simulink model "stepResponseDDR"  (R2021a)
settings: Solver=VariableStepAuto  StartTime=0.0  StopTime=20  RelTol=1e-3
model workspace (MAT data in the model file):
  Velocity = 2
  axleLength = 0.1
  radius = 0.02
libraries: simulink x2, robotmobilelib x1, pid_lib x1
settings Model: NumberOfSteps=10  EnablePacing=on  PacingRate=6  Creator=yellu  LastModifiedBy=yellu

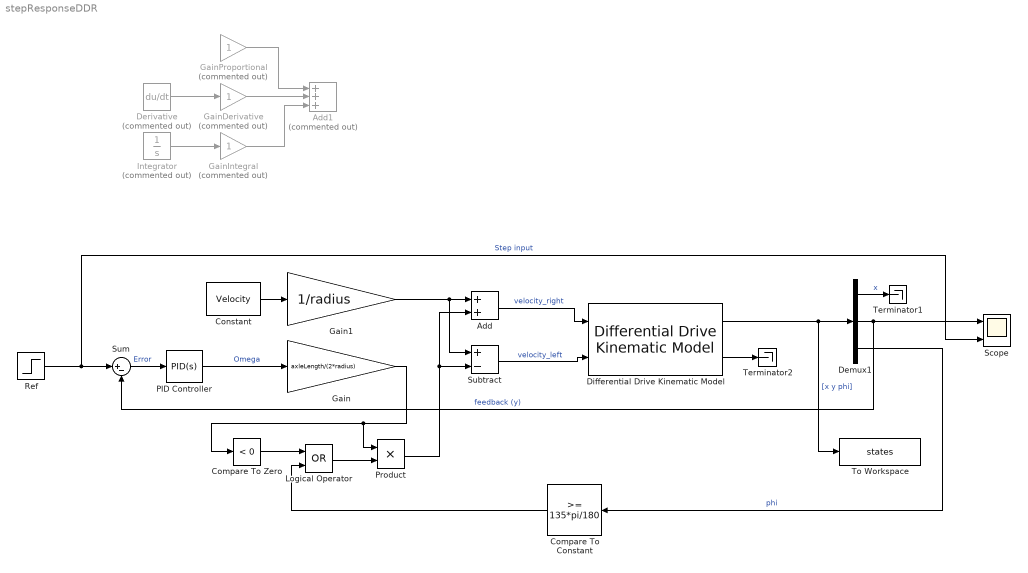
== system stepResponseDDR ==
  Add : Sum
  Add1 : Sum  Commented=on  Inputs=+++
  Compare To Constant : simulink/Logic and Bit Operations/Compare To Constant  relop=>=  const=135*pi/180  OutDataTypeStr=boolean
  Compare To Zero : simulink/Logic and Bit Operations/Compare To Zero  relop=<  OutDataTypeStr=boolean
  Constant : Constant  Value=Velocity
  Demux1 : Demux  Outputs=3
  Derivative : Derivative  Commented=on
  Differential Drive Kinematic Model : robotmobilelib/Differential Drive Kinematic Model  VehicleInputs=Wheel Speeds  WheelRadius=radius  WheelSpeedRange=[-inf inf]  TrackWidth=axleLength  InitialState=[0 0 180*pi/180]  SimulateUsing=Interpreted execution
      settings: SourceProductBaseCode=RO
  Gain : Gain  Gain=axleLength/(2*radius)
  Gain1 : Gain  Gain=1/radius
  GainDerivative : Gain  Commented=on
  GainIntegral : Gain  Commented=on
  GainProportional : Gain  Commented=on
  Integrator : Integrator  Commented=on
  Logical Operator : Logic  Operator=OR  AllPortsSameDT=off  OutDataTypeStr=boolean
  PID Controller : pid_lib/PID Controller  Controller=PID  Form=Parallel  TimeDomain=Continuous-time  UseExternalTs=off  SampleTime=-1  IntegratorMethod=Forward Euler  FilterMethod=Forward Euler  ControllerParametersSource=internal  P=0.5  I=0  D=0.8  UseFilter=on  N=100  TunerSelectOption=Transfer Function Based (PID Tuner App)  InitialConditionSource=internal  InitialConditionForIntegrator=0  InitialConditionForFilter=0  DifferentiatorICPrevScaledInput=0  ExternalReset=none  TrackingMode=off  Kt=1  LimitOutput=on  SatLimitsSource=internal  UpperSaturationLimit=4.48  LowerSaturationLimit=-4.48  LinearizeAsGain=on  AntiWindupMode=clamping  Kb=1  POutMin=[]  POutMax=[]  IOutMin=[]  IOutMax=[]  DOutMin=[]  DOutMax=[]  NOutMin=[]  NOutMax=[]  SumOutMin=[]  SumOutMax=[]  SaturationOutMin=[]  SaturationOutMax=[]  PParamMin=[]  PParamMax=[]  IParamMin=[]  IParamMax=[]  DParamMin=[]  DParamMax=[]  NParamMin=[]  NParamMax=[]  KbParamMin=[]  KbParamMax=[]  KtParamMin=[]  KtParamMax=[]  KbOutMin=[]  KbOutMax=[]  KtOutMin=[]  KtOutMax=[]  IntegratorOutMin=[]  IntegratorOutMax=[]  FilterOutMin=[]  FilterOutMax=[]  SumI1OutMin=[]  SumI1OutMax=[]  SumI2OutMin=[]  SumI2OutMax=[]  SumI3OutMin=[]  SumI3OutMax=[]  SumI4OutMin=[]  SumI4OutMax=[]  SumDOutMin=[]  SumDOutMax=[]  DifferentiatorOutMin=[]  DifferentiatorOutMax=[]  FilterDiffOutCoefMin=[]  FilterDiffOutCoefMax=[]  ReciprocalOutMin=[]  ReciprocalOutMax=[]  SumDenOutMin=[]  SumDenOutMax=[]  SumNumOutMin=[]  SumNumOutMax=[]  DivideOutMin=[]  DivideOutMax=[]  UdiffTsProdOutMin=[]  UdiffTsProdOutMax=[]  NTsProdOutMin=[]  NTsProdOutMax=[]  UintegralTsProdOutMin=[]  UintegralTsProdOutMax=[]  UngainTsProdOutMin=[]  UngainTsProdOutMax=[]  IntegratorContinuousStateAttributes=''  IntegratorStateMustResolveToSignalObject=off  IntegratorRTWStateStorageClass=Auto  FilterContinuousStateAttributes=''  FilterStateMustResolveToSignalObject=off  FilterRTWStateStorageClass=Auto  ParallelPVariant=InternalParameters  IdealPVariant=Disabled  IVariant=InternalParameters  DVariant=InternalParameters  IntegratorVariant=Continuous  SatVariant=Enabled  AWVariant=ContClampingParallel  PCopyVariant=Disabled  TRVariant=Disabled  FdbkBlocksVariant=Forward  IdealPFdbkVariant=Disabled  SatFdbkVariant=Disabled  DerivativeFilterVariant=ContFilter  NVariant=InternalParameters  NCopyVariant=Disabled  FilterICVariant=InternalICsFilter  IntegratorICVariant=InternalICs  ExternalResetVariant=Disabled  TRSumVariant=Passthrough  SumFdbkVariant=Disabled  SumVariant=Sum_PID  TsampFilterVariant=InternalTs  TsampNgainVariant=Passthrough  TsampIntegralVariant=Passthrough  ExternalSaturationOutDataTypeStr=Inherit: Same as second input  InitialConditionSetting=Output
  Product : Product
  Ref : Step  Time=3  After=5  SampleTime=0  VectorParams1D=off
  Scope : Scope  NumInputPorts=2
  Subtract : Sum  Inputs=+-
  Sum : Sum  Inputs=|+-
  Terminator1 : Terminator
  Terminator2 : Terminator
  To Workspace : ToWorkspace  VariableName=states  SampleTime=-1
  wires:
  Constant/1 -> Gain1/1
  Gain1/1 -> Subtract/1, Add/1
  Add/1 -> Differential Drive Kinematic Model/1  "velocity_right"
  Subtract/1 -> Differential Drive Kinematic Model/2  "velocity_left"
  GainProportional/1 -> Add1/1
  Ref/1 -> Scope/2, Sum/1  "Step input"
  Differential Drive Kinematic Model/1 -> To Workspace/1, Demux1/1  "[x y phi]"
  GainIntegral/1 -> Add1/3
  GainDerivative/1 -> Add1/2
  Derivative/1 -> GainDerivative/1
  Integrator/1 -> GainIntegral/1
  PID Controller/1 -> Gain/1  "Omega"
  Demux1/2 -> Sum/2, Scope/1  "feedback (y)"
  Demux1/1 -> Terminator1/1  "x"
  Sum/1 -> PID Controller/1  "Error"
  Differential Drive Kinematic Model/2 -> Terminator2/1
  Compare To Constant/1 -> Logical Operator/2
  Demux1/3 -> Compare To Constant/1  "phi"
  Gain/1 -> Product/1, Compare To Zero/1
  Compare To Zero/1 -> Logical Operator/1
  Product/1 -> Add/2, Subtract/2
  Logical Operator/1 -> Product/2
